simulink model "sim_tcyb_2025_obs"  (R2020a)
settings: Solver=ode4  StartTime=0.0  StopTime=30.0  FixedStep=0.01  RelTol=1e-3
values from neighbouring files (symbols this model uses):
  epst = 0.01    [init_tcyb_2025_obs.m]
  k01 = 0.6    [init_tcyb_2025_obs.m]
  k02 = 4    [init_tcyb_2025_obs.m]
  k03 = 0.6    [init_tcyb_2025_obs.m]
  k04 = 4    [init_tcyb_2025_obs.m]
  kai_1_t = 0.02    [init_tcyb_2025_obs.m]
  kai_3_t = 0.1    [init_tcyb_2025_obs.m]
  Mii = diag([1;0;0;0;1])    [init_tcyb_2025_obs.m]
  pos0 = zeros(3, 1)    [init_tcyb_2025_obs.m]
  PZ0 = P0(3)    [init_tcyb_2025_obs.m]
  PZ1 = 10    [init_tcyb_2025_obs.m]
  R0 = 4    [init_tcyb_2025_obs.m]
  R1 = 8    [init_tcyb_2025_obs.m]
  Rx2 = 10    [init_tcyb_2025_obs.m]
  Ry2 = 6    [init_tcyb_2025_obs.m]
  Rz2 = 4    [init_tcyb_2025_obs.m]
  T0 = 6.0    (= 6)    [init_tcyb_2025_obs.m]
  T1 = tseq1    (= 10)    [init_tcyb_2025_obs.m]
  T12 = tseq1 + tseq12    (= 20)    [init_tcyb_2025_obs.m]
  T2 = tseq1 + tseq12 + tseq2    (= 30)    [init_tcyb_2025_obs.m]
  theta0 = ( 2 / 5 ) * pi    (= 1.25663706144)    [init_tcyb_2025_obs.m]
  vel0 = zeros(3, 1)    [init_tcyb_2025_obs.m]
  Wij = [0,0,1,0,0;              0,0,1,1,0;              1,0,0,0,1;              0,1,1,0,0;              0,0,1,0,0]    [init_tcyb_2025_obs.m]
  X1 = 8    [init_tcyb_2025_obs.m]
  X2 = 2    [init_tcyb_2025_obs.m]
  X3 = 3    [init_tcyb_2025_obs.m]
  Y1 = 10    [init_tcyb_2025_obs.m]
  Y2 = 2    [init_tcyb_2025_obs.m]
  Y3 = 4    [init_tcyb_2025_obs.m]
  Z1 = 4    [init_tcyb_2025_obs.m]
  Z2 = -6    [init_tcyb_2025_obs.m]
  Z3 = 2    [init_tcyb_2025_obs.m]
(part 2 of 2)

== matlab function sim_tcyb_2025_obs/leader control input ==
  data: t input; u0 output; T1 input; T2 input; R0 input; R1 input; Rx2 input; Ry2 input; Rz2 input
function u0  = fcn(t, T1, T2, R0, R1, Rx2, Ry2, Rz2)
%%%% 给出领导者参考加速度控制输入
u0 = zeros(3, 1);

if t <= ( T1 + 1e-05 )
    u0(1, 1) = - ( 4 * pi * sin( ( 2 * pi * ( t - 0 ) ) / ( 0 - T1 ) ) * ( R0 - R1 ) ) / ( ( 0 - T1 ) ^ 2 ) ...
                        - ( 4 * ( pi ^ 2 ) * cos( ( 2 * pi * ( t - 0 ) ) / ( 0 - T1 ) ) ...
                        * ( R0 + ( ( R0 - R1 ) * ( t - 0 ) ) / ( 0 - T1 ) ) ) / ( ( 0 - T1 ) ^ 2 );
    u0(2, 1) = ( 4 * pi * cos( ( 2 * pi * ( t - 0 ) ) / ( 0 - T1 ) ) * ( R0 - R1 ) ) / ( ( 0 - T1 ) ^ 2 ) ...
                        - ( 4 * ( pi ^ 2 ) * sin( ( 2 * pi * ( t - 0 ) ) / ( 0 - T1 ) ) ...
                        * ( R0 + ( ( R0 - R1 ) * ( t - 0 ) ) / ( 0 - T1 ) ) ) / ( ( 0 - T1 ) ^ 2 );
    u0(3, 1) = 0;
else
    u0(1, 1) = ( 4 * Rx2 * ( pi ^ 2 ) * cos( ( 2 * pi * ( t - T1 ) ) / ( T1 - T2 ) ) ) / ( ( T1 - T2 ) ^ 2 );
    u0(2, 1) = - ( 16 * Ry2 * ( pi ^ 2 ) * sin( ( 4 * pi * ( t - T1 ) ) / ( T1 - T2 ) ) ) / ( ( T1 - T2 ) ^ 2 );
    u0(3, 1) = ( 16 * Rz2 * ( pi ^ 2 ) * sin( ( 4 * pi * ( t - T1 ) ) / ( T1 - T2 ) ) ) / ( ( T1 - T2 ) ^ 2 );
end
